simulink model "wahadlo_model_matematyczny_2015a"  (R2015a)
settings: Solver=ode45  SolverMode=SingleTasking  StartTime=0.0  StopTime=10.0  RelTol=1e-3
values from neighbouring files (symbols this model uses):
  b = a_1 * a_2    [Wahadlo_setup.m]
  f_c = 1.0942    [clean_pendulum_setup.m]
  g = 9.8101    [Wahadlo_setup.m]    (also in clean_pendulum_setup.m = 9.81)
  mL = m * L    [Wahadlo_setup.m]
undefined symbols (not defined in the file or in its folder): a1, a2, k1, k2, k3
settings Model: CovMetricSettings=dwe  CovHtmlReporting=off  covSaveCumulativeToWorkspaceVar=off  CovSaveSingleToWorkspaceVar=off  CovExternalEMLEnable=on  Creator=tomas  LastModifiedBy=tomas
settings DataIOCC: LimitDataPoints=off  SaveFormat=Dataset  ReturnWorkspaceOutputs=on
settings DebuggingCC: SFUnexpectedBacktrackingDiag=error  SFNoUnconditionalDefaultTransitionDiag=error
settings HardwareCC: ProdBitPerPointer=64  ProdLargestAtomicFloat=Float  ProdIntDivRoundTo=Zero  ProdEndianess=LittleEndian  ProdHWDeviceType=Specified
settings ModelReferenceCC: PropagateSignalLabelsOutOfModel=on
settings SFSimCC: SimUseLocalCustomCode=on
settings RTWCC: RTWUseLocalCustomCode=on
settings GRTTargetCC: TargetLangStandard=C99 (ISO)

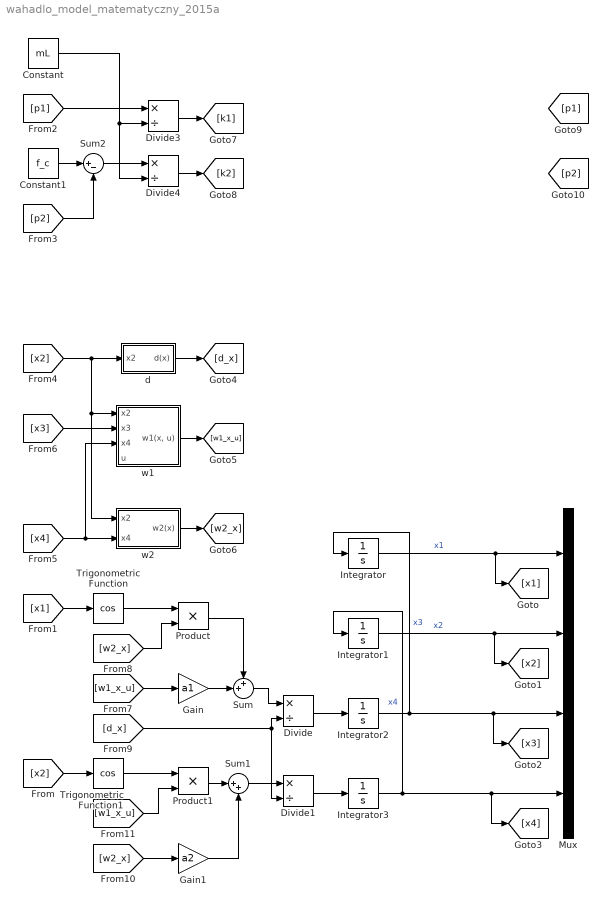
== system wahadlo_model_matematyczny_2015a ==
  Constant : Constant  Value=mL
  Constant1 : Constant  Value=f_c
  Divide{,1,3..4} (4 alike) : Product  Inputs=*/
  Gain : Gain  Gain=a1
  Gain1 : Gain  Gain=a2
  Integrator{,1..3} (4 alike) : Integrator
  Mux : Mux
  Product : Product
  Product1 : Product
  Sum : Sum  Inputs=++|
  Sum1 : Sum  Inputs=|++
  Sum2 : Sum  Inputs=|+-
  Trigonometric Function : Trigonometry  Operator=cos
  Trigonometric Function1 : Trigonometry  Operator=cos
  d : Subsystem
  w1 : Subsystem
  w2 : Subsystem
  wires:
  Integrator/1 -> [x1], Mux/1  "x1"
  Integrator1/1 -> [x2], Mux/2  "x2"
  Integrator2/1 -> Integrator/1, [x3], Mux/3  "x3"
  Integrator3/1 -> Integrator1/1, [x4], Mux/4  "x4"
  Trigonometric Function/1 -> Product/1
  [x2] -> Trigonometric Function1/1
  Divide/1 -> Integrator2/1
  Sum/1 -> Divide/1
  Gain/1 -> Sum/2
  Product/1 -> Sum/1
  w2/1(w2(x)) -> [w2_x]
  w1/1("w1(x, u)") -> [w1_x_u]
  d/1(d(x)) -> [d_x]
  [x2] -> w2/1(x2), w1/1(x2), d/1(x2)
  [x4] -> w1/3(x4), w2/2(x4)
  [x3] -> w1/2(x3)
  [w1_x_u] -> Gain/1
  [w2_x] -> Product/2
  [d_x] -> Divide1/2, Divide/2
  [w1_x_u] -> Product1/2
  Trigonometric Function1/1 -> Product1/1
  [x1] -> Trigonometric Function/1
  [w2_x] -> Gain1/1
  Product1/1 -> Sum1/1
  Sum1/1 -> Divide1/1
  Gain1/1 -> Sum1/2
  Divide1/1 -> Integrator3/1
  Divide3/1 -> [k1]
  Divide4/1 -> [k2]
  [p1] -> Divide3/1
  Constant/1 -> Divide3/2, Divide4/2
  Sum2/1 -> Divide4/1
  [p2] -> Sum2/2
  Constant1/1 -> Sum2/1

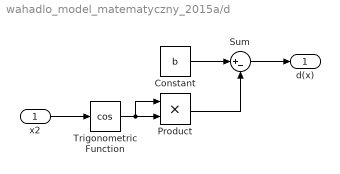
== system wahadlo_model_matematyczny_2015a/d ==
  x2 : Inport
  Constant : Constant  Value=b
  Product : Product
  Sum : Sum  Inputs=|+-
  Trigonometric Function : Trigonometry  Operator=cos
  d(x) : Outport
  wires:
  Trigonometric Function/1 -> Product/1, Product/2
  Product/1 -> Sum/2
  x2/1 -> Trigonometric Function/1
  Constant/1 -> Sum/1
  Sum/1 -> d(x)/1

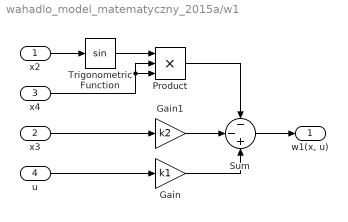
== system wahadlo_model_matematyczny_2015a/w1 ==
  x2 : Inport
  x3 : Inport  Port=2
  x4 : Inport  Port=3
  u : Inport  Port=4
  Gain : Gain  Gain=k1
  Gain1 : Gain  Gain=k2
  Product : Product  Inputs=3
  Sum : Sum  Inputs=--+
  Trigonometric Function : Trigonometry
  "w1(x, u)" : Outport
  wires:
  Gain/1 -> Sum/3
  Product/1 -> Sum/1
  Gain1/1 -> Sum/2
  Sum/1 -> "w1(x, u)"/1
  x3/1 -> Gain1/1
  x2/1 -> Trigonometric Function/1
  Trigonometric Function/1 -> Product/1
  x4/1 -> Product/3, Product/2
  u/1 -> Gain/1

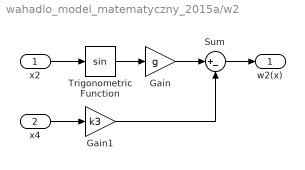
== system wahadlo_model_matematyczny_2015a/w2 ==
  x2 : Inport
  x4 : Inport  Port=2
  Gain : Gain  Gain=g
  Gain1 : Gain  Gain=k3
  Sum : Sum  Inputs=|+-
  Trigonometric Function : Trigonometry
  w2(x) : Outport
  wires:
  Trigonometric Function/1 -> Gain/1
  x2/1 -> Trigonometric Function/1
  x4/1 -> Gain1/1
  Gain/1 -> Sum/1
  Gain1/1 -> Sum/2
  Sum/1 -> w2(x)/1
